simulink model "F16_fcs"  (Simulink 7.3)
settings: Solver=ode3  StartTime=0.0  StopTime=simtime  FixedStep=0.02  RelTol=1e-3
undefined symbols (not defined in the file or in its folder): alpha_trim, da_trim, del_trim, der_trim, dlef_trim, dr_trim, Earth, f16, fi_flag_Simulink, m, mlu, roll_trim, s, V_trim, WGS84, yaw_trim
libraries: simulink_extras x16, aerolibfltsims x3, aerolibtransform2 x3, simulink x2, aerolibanimutils x2, aerolibconvert2 x2, aerolibconvert x1, aerolibutil x1
settings Model: Creator=larssonneveldt  LastModifiedBy=Administrator
settings DataIOCC: SignalLoggingName=sigsOut
settings OptimizationCC: InlineInvariantSignals=on  InitFltsAndDblsToZero=on
settings DebuggingCC: SignalResolutionControl=TryResolveAllWithWarning  SolverPrmCheckMsg=none  MultiTaskDSMMsg=warning  MultiTaskCondExecSysMsg=none  StrictBusMsg=None
settings HardwareCC: TargetHWDeviceType=32-bit Generic  TargetUnknown=on  ProdEqTarget=off
settings RTWCC: IncludeERTFirstTime=on
settings GRTTargetCC: TargetFcnLib=ansi_tfl_tmw.mat

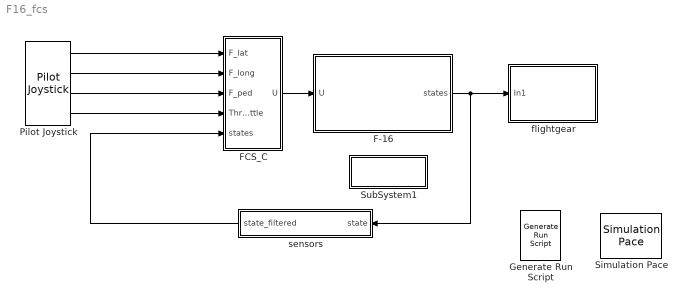
== system F16_fcs ==
  F-16 : Subsystem
      mask Display: image(imread('aerodata/f16.jpg'))
  FCS_C : Subsystem
  Generate Run Script : aerolibfltsims/Generate Run Script  DialogController=Aeroblks.DDGSource  SystemSampleTime=-1  OutputFileName=runfg.bat  FlightGearBaseDirectory=D:\Program Files\FlightGear  GeometryModelName=f16-mlu  DestinationPort=5502  AirportId=KSFO  RunwayId=10L  InitialAltitude=1000  InitialHeading=113  OffsetDistance=4.72  OffsetAzimuth=0  GenerateFile=off
  Pilot Joystick : aerolibanimutils/Pilot Joystick  JoystickID=Joystick1  OutputConfiguration=FourAxis  SampleTime=1/50
  Simulation Pace : aerolibanimutils/Simulation Pace  SimulationPace=1  SleepMode=MATLAB Thread  OutputPaceError=off  SampleTime=-1
      settings: AttributesFormatString=%<SimulationPace> sec/sec
  SubSystem1 : Subsystem
      settings: OpenFcn=edit(fullfile(cd,'F16_dyn.c'))
      mask Display: disp('F16_dyn.c');
  flightgear : Subsystem
  sensors : Subsystem
  wires:
  Pilot Joystick/1 -> FCS_C/1(F_lat)
  Pilot Joystick/2 -> FCS_C/2(F_long)
  Pilot Joystick/4 -> FCS_C/4(Throttle)
  sensors/1(state_filtered) -> FCS_C/5(states)
  F-16/1(states) -> flightgear/1(In1), sensors/1(state)
  FCS_C/1(U) -> F-16/1(U)
  Pilot Joystick/3 -> FCS_C/3(F_ped)

== system F16_fcs/F-16 ==
  U : Inport
  F-16 dynamics : S-Function  FunctionName=F16_dyn  Parameters=init_x  EnableBusSupport=off
      mask Display: image(imread('aerodata/f16.jpg'))
  LEF : Subsystem
      mask Display: port_label('output', 1, 'dlef')
  Mux : Mux  Inputs=2
  fi_flag : Constant  Value=fi_flag_Simulink  OutDataType=sfix(16)  OutScaling=2^0
  states : Outport
  wires:
  fi_flag/1 -> F-16 dynamics/3
  LEF/1("delta_lef ") -> F-16 dynamics/2
  U/1 -> F-16 dynamics/1
  F-16 dynamics/1 -> LEF/1(state), Mux/1
  F-16 dynamics/2 -> Mux/2
  Mux/1 -> states/1

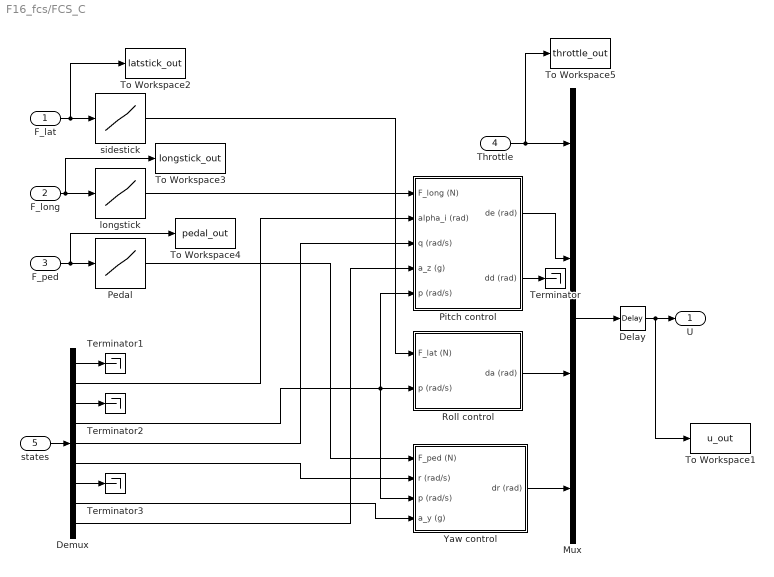
== system F16_fcs/FCS_C ==
  F_lat : Inport  OutDataType=sfix(16)  OutScaling=2^0
  F_long : Inport  Port=2  OutDataType=sfix(16)  OutScaling=2^0
  F_ped : Inport  Port=3  OutDataType=sfix(16)  OutScaling=2^0
  Throttle : Inport  Port=4  OutDataType=sfix(16)  OutScaling=2^0
  states : Inport  Port=5  OutDataType=sfix(16)  OutScaling=2^0
  Delay : TransportDelay  DelayTime=0.02
  Demux : Demux  Outputs=[2 1 3 1 1 1 4 1 1]
  Mux : Mux
  Pedal : Lookup  InputValues=[-1 -0.5 0.2 0.2 0.5 1]  Table=[-520 -70 0 0 70 520]  OutDataType=sfix(16)  OutScaling=2^0
  Pitch control : Subsystem
  Roll control : Subsystem
  Terminator{,1..3} (4 alike) : Terminator
  To Workspace1 : ToWorkspace  VariableName=u_out  SampleTime=-1  SaveFormat=Structure With Time
  To Workspace2 : ToWorkspace  VariableName=latstick_out  SampleTime=-1  SaveFormat=Structure With Time
  To Workspace3 : ToWorkspace  VariableName=longstick_out  SampleTime=-1  SaveFormat=Structure With Time
  To Workspace4 : ToWorkspace  VariableName=pedal_out  SampleTime=-1  SaveFormat=Structure With Time
  To Workspace5 : ToWorkspace  VariableName=throttle_out  SampleTime=-1  SaveFormat=Structure With Time
  Yaw control : Subsystem
  longstick : Lookup  InputValues=[-1,-0.5,-0.125,0.125,0.5,1]  Table=[-60,-20,0,0,30,160]  OutDataType=sfix(16)  OutScaling=2^0
  sidestick : Lookup  InputValues=[-1,-0.5,-0.2,0.2,0.5,1]  Table=[-80,-20,0,0,20,80]  OutDataType=sfix(16)  OutScaling=2^0
  U : Outport  OutDataType=sfix(16)  OutScaling=2^0
  wires:
  Pitch control/2(dd (rad)) -> Terminator/1
  Pitch control/1(de (rad)) -> Mux/2
  Yaw control/1(dr (rad)) -> Mux/4
  Mux/1 -> Delay/1
  Throttle/1 -> Mux/1, To Workspace5/1
  F_ped/1 -> Pedal/1, To Workspace4/1
  states/1 -> Demux/1
  Demux/1 -> Terminator1/1
  Demux/3 -> Terminator2/1
  Demux/7 -> Terminator3/1
  Demux/2 -> Pitch control/2(alpha_i (rad))
  Demux/4 -> Roll control/2(p (rad/s)), Pitch control/5(p (rad/s)), Yaw control/3(p (rad/s))
  Demux/5 -> Pitch control/3(q (rad/s))
  Demux/6 -> Yaw control/2(r (rad/s))
  F_long/1 -> longstick/1, To Workspace3/1
  F_lat/1 -> sidestick/1, To Workspace2/1
  Delay/1 -> U/1, To Workspace1/1
  Roll control/1(da (rad)) -> Mux/3
  Demux/9 -> Pitch control/4(a_z (g))
  Demux/8 -> Yaw control/4(a_y (g))
  sidestick/1 -> Roll control/1(F_lat (N))
  longstick/1 -> Pitch control/1(F_long (N))
  Pedal/1 -> Yaw control/1(F_ped (N))

== system F16_fcs/SubSystem1 ==

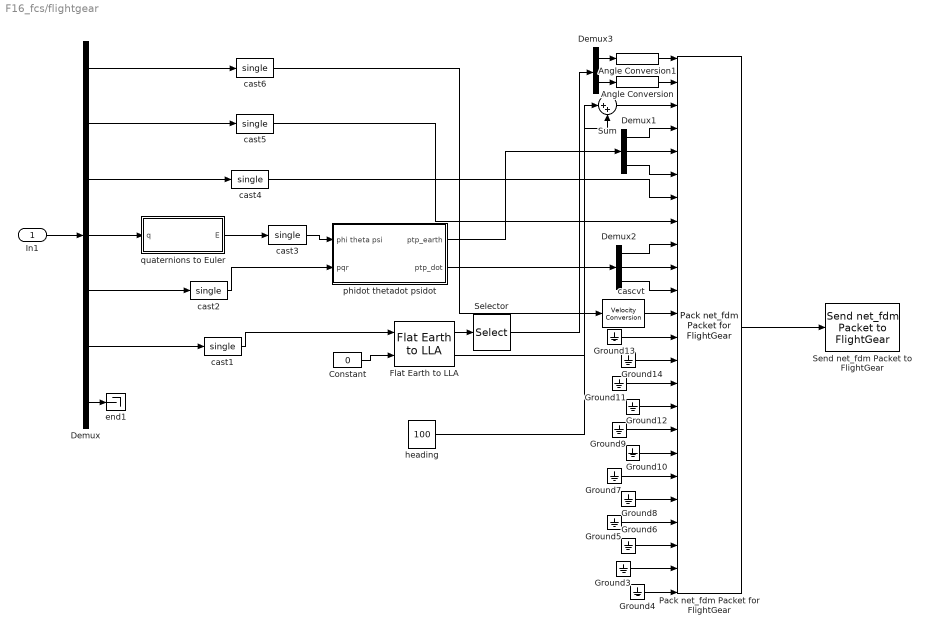
== system F16_fcs/flightgear ==
  In1 : Inport
  Angle Conversion : aerolibconvert2/Angle Conversion  SystemSampleTime=-1  IU=deg  OU=rad
  Angle Conversion1 : aerolibconvert2/Angle Conversion  SystemSampleTime=-1  IU=deg  OU=rad
  Constant : Constant  Value=0  OutDataType=sfix(16)  OutScaling=2^0
  Demux : Demux  Outputs=[1 1 1 4 3 3 3]
  Demux1 : Demux  Outputs=3
  Demux2 : Demux  Outputs=3
  Demux3 : Demux  Outputs=2
  Flat Earth to LLA : aerolibtransform2/Flat Earth to LLA  SystemSampleTime=-1  units=Metric (MKS)  ptype=Earth (WGS84)  F=1/298.257223563  R=6378137  LL0=[37.7889 -122.4778]  psi=0
  Ground{3..14} (12 alike) : Ground
  Pack net_fdm Packet for FlightGear : aerolibfltsims/Pack net_fdm Packet for FlightGear  FlightGearVersion=v0.9.10  ShowPositionAttitudeInputs=on  ShowVelocityAccelerationInputs=on  ShowControlSurfacePositionInputs=off  ShowEngineFuelInputs=off  ShowLandingGearInputs=off  ShowEnvironmentInputs=off  SampleTime=-1
  Selector : Selector  InputPortWidth=2  IndexOptions=Index vector (dialog)  Indices=[2 1]  OutputSizes=1
  Send net_fdm Packet to FlightGear : aerolibfltsims/Send net_fdm Packet to FlightGear  DestinationIpAddress=127.0.0.1  DestinationPort=5502  LocalIpPort=-1  SampleTime=-1
  Sum : Sum  Inputs=|++  OutDataType=sfix(16)  OutScaling=2^0
  cascvt : aerolibconvert/Velocity Conversion  SystemSampleTime=-1  IU=m/s  OU=kts
  cast{1..6} (6 alike) : DataTypeConversion  OutDataTypeMode=single  OutDataType=sfix(16)  OutScaling=2^0  OutDataTypeStr=single  SaturateOnIntegerOverflow=on
  end1 : Terminator
  heading : Constant  Value=100  OutDataType=sfix(16)  OutScaling=2^0
  phidot thetadot psidot : Subsystem
  quaternions to Euler : Subsystem
  wires:
  Ground3/1 -> Pack net_fdm Packet for FlightGear/23
  Ground4/1 -> Pack net_fdm Packet for FlightGear/24
  Ground5/1 -> Pack net_fdm Packet for FlightGear/21
  Ground6/1 -> Pack net_fdm Packet for FlightGear/22
  Ground7/1 -> Pack net_fdm Packet for FlightGear/19
  Ground8/1 -> Pack net_fdm Packet for FlightGear/20
  Ground9/1 -> Pack net_fdm Packet for FlightGear/17
  Ground10/1 -> Pack net_fdm Packet for FlightGear/18
  Ground11/1 -> Pack net_fdm Packet for FlightGear/15
  Ground12/1 -> Pack net_fdm Packet for FlightGear/16
  Ground13/1 -> Pack net_fdm Packet for FlightGear/13
  Ground14/1 -> Pack net_fdm Packet for FlightGear/14
  Pack net_fdm Packet for FlightGear/1 -> Send net_fdm Packet to FlightGear/1
  cascvt/1 -> Pack net_fdm Packet for FlightGear/12
  In1/1 -> Demux/1
  Demux/1 -> cast6/1
  Demux/2 -> cast5/1
  Demux1/1 -> Pack net_fdm Packet for FlightGear/4
  Demux1/3 -> Pack net_fdm Packet for FlightGear/6
  Demux/3 -> cast4/1
  Demux2/1 -> Pack net_fdm Packet for FlightGear/9
  Demux2/2 -> Pack net_fdm Packet for FlightGear/10
  Demux/5 -> cast2/1
  Demux2/3 -> Pack net_fdm Packet for FlightGear/11
  Demux1/2 -> Pack net_fdm Packet for FlightGear/5
  phidot thetadot psidot/1(ptp_earth) -> Demux1/1
  phidot thetadot psidot/2(ptp_dot) -> Demux2/1
  Demux/6 -> cast1/1
  Constant/1 -> Flat Earth to LLA/2
  Flat Earth to LLA/1 -> Selector/1
  Selector/1 -> Demux3/1
  Demux3/1 -> Angle Conversion1/1
  Demux3/2 -> Angle Conversion/1
  cast1/1 -> Flat Earth to LLA/1
  cast2/1 -> phidot thetadot psidot/2(pqr)
  cast3/1 -> phidot thetadot psidot/1(phi theta psi)
  cast4/1 -> Pack net_fdm Packet for FlightGear/7
  cast5/1 -> Pack net_fdm Packet for FlightGear/8
  cast6/1 -> cascvt/1
  Flat Earth to LLA/2 -> Sum/1
  Sum/1 -> Pack net_fdm Packet for FlightGear/3
  Angle Conversion/1 -> Pack net_fdm Packet for FlightGear/2
  Angle Conversion1/1 -> Pack net_fdm Packet for FlightGear/1
  heading/1 -> Sum/2
  quaternions to Euler/1(E) -> cast3/1
  Demux/4 -> quaternions to Euler/1(q)
  Demux/7 -> end1/1

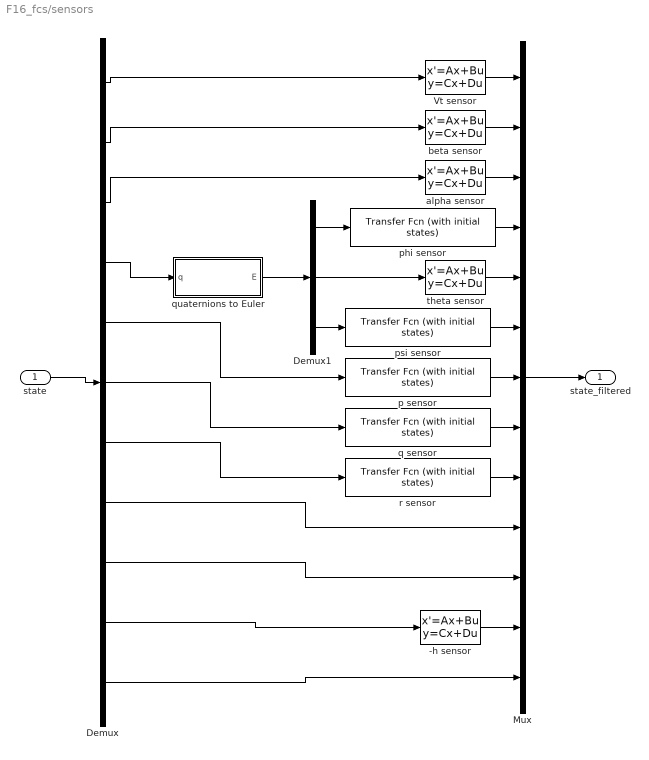
== system F16_fcs/sensors ==
  state : Inport
  -h sensor : StateSpace  A=-50  B=50  D=0  X0=alpha_trim
  Demux : Demux  Outputs=[ones(1,3) 4 ones(1,6) 3]
  Demux1 : Demux  Outputs=3
  Mux : Mux  Inputs=[ones(1,12) 3]
  Vt sensor : StateSpace  A=-50  B=50  D=0  X0=V_trim
  alpha sensor : StateSpace  A=-50  B=50  D=0  X0=alpha_trim
  beta sensor : StateSpace  A=-50  B=50  D=0
  p sensor : simulink_extras/Additional Linear/Transfer Fcn (with initial states)  SystemSampleTime=-1  N=[0.0001903 0.005346 1]  D=[0.0004942 0.03082 1]  X0=[0 0]
  phi sensor : simulink_extras/Additional Linear/Transfer Fcn (with initial states)  SystemSampleTime=-1  N=[1]  D=[0.00104 0.0323 1]  X0=[0 0]
  psi sensor : simulink_extras/Additional Linear/Transfer Fcn (with initial states)  SystemSampleTime=-1  N=[1]  D=[0.00104 0.0323 1]  X0=[0 0]
  q sensor : simulink_extras/Additional Linear/Transfer Fcn (with initial states)  SystemSampleTime=-1  N=[0.0001903 0.005346 1]  D=[0.0004942 0.03082 1]  X0=[0 0]
  quaternions to Euler : Subsystem
  r sensor : simulink_extras/Additional Linear/Transfer Fcn (with initial states)  SystemSampleTime=-1  N=[0.0001903 0.005346 1]  D=[0.0004942 0.03082 1]  X0=[0 0]
  theta sensor : StateSpace  A=-50  B=50  D=0  X0=alpha_trim
  state_filtered : Outport
  wires:
  Mux/1 -> state_filtered/1
  state/1 -> Demux/1
  r sensor/1 -> Mux/9
  q sensor/1 -> Mux/8
  p sensor/1 -> Mux/7
  psi sensor/1 -> Mux/6
  phi sensor/1 -> Mux/4
  alpha sensor/1 -> Mux/3
  beta sensor/1 -> Mux/2
  Vt sensor/1 -> Mux/1
  Demux1/1 -> phi sensor/1
  Demux1/2 -> theta sensor/1
  Demux1/3 -> psi sensor/1
  -h sensor/1 -> Mux/12
  quaternions to Euler/1(E) -> Demux1/1
  theta sensor/1 -> Mux/5
  Demux/1 -> Vt sensor/1
  Demux/2 -> beta sensor/1
  Demux/3 -> alpha sensor/1
  Demux/4 -> quaternions to Euler/1(q)
  Demux/5 -> p sensor/1
  Demux/6 -> q sensor/1
  Demux/7 -> r sensor/1
  Demux/8 -> Mux/10
  Demux/9 -> Mux/11
  Demux/10 -> -h sensor/1
  Demux/11 -> Mux/13

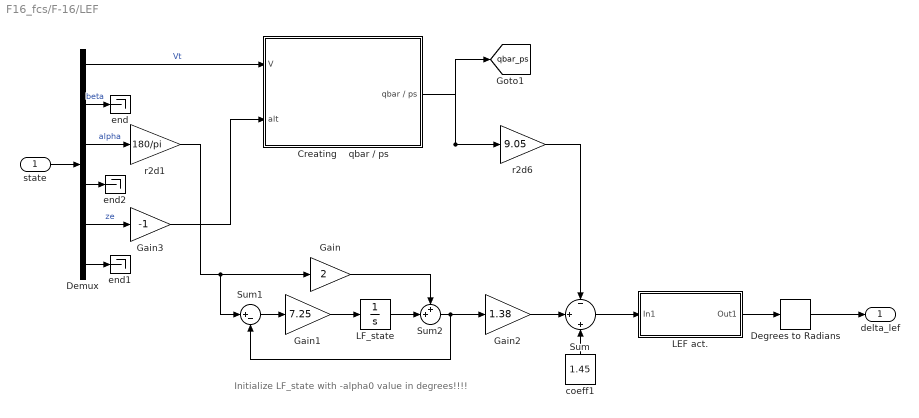
== system F16_fcs/F-16/LEF ==
  note: Initialize LF_state with -alpha0 value in degrees!!!!
  state : Inport  OutDataType=sfix(16)  OutScaling=2^0
  Creating    qbar / ps : Subsystem
  Degrees to Radians : simulink_extras/Transformations/Degrees to Radians  SystemSampleTime=-1
  Demux : Demux  Outputs=[1 1 1 9 1 1]
  Gain : Gain  Gain=2  ParameterDataType=sfix(16)  ParameterScaling=2^0  OutDataType=sfix(16)  OutScaling=2^0  SaturateOnIntegerOverflow=on  OutDataTypeStr=Inherit: Same as input  ParamDataTypeStr=Inherit: Same as input
  Gain1 : Gain  Gain=7.25  ParameterDataType=sfix(16)  ParameterScaling=2^0  OutDataType=sfix(16)  OutScaling=2^0  SaturateOnIntegerOverflow=on  OutDataTypeStr=Inherit: Same as input  ParamDataTypeStr=Inherit: Same as input
  Gain2 : Gain  Gain=1.38  ParameterDataType=sfix(16)  ParameterScaling=2^0  OutDataType=sfix(16)  OutScaling=2^0  SaturateOnIntegerOverflow=on  OutDataTypeStr=Inherit: Same as input  ParamDataTypeStr=Inherit: Same as input
  Gain3 : Gain  Gain=-1  ParameterDataType=sfix(16)  ParameterScaling=2^0  OutDataType=sfix(16)  OutScaling=2^0  SaturateOnIntegerOverflow=on  OutDataTypeStr=Inherit: Same as input  ParamDataTypeStr=Inherit: Same as input
  LEF act. : Subsystem
  LF_state : Integrator  InitialCondition=-alpha_trim*180/pi
  Sum : Sum  Inputs=-|+|+  OutDataType=sfix(16)  OutScaling=2^0  SaturateOnIntegerOverflow=on  InputSameDT=on  OutDataTypeStr=Inherit: Same as first input
  Sum1 : Sum  Inputs=|+-  OutDataType=sfix(16)  OutScaling=2^0  SaturateOnIntegerOverflow=on  InputSameDT=on  OutDataTypeStr=Inherit: Same as first input
  Sum2 : Sum  Inputs=++|  OutDataType=sfix(16)  OutScaling=2^0  SaturateOnIntegerOverflow=on  InputSameDT=on  OutDataTypeStr=Inherit: Same as first input
  coeff1 : Constant  Value=1.45  OutDataType=sfix(16)  OutScaling=2^0
  end : Terminator
  end1 : Terminator
  end2 : Terminator
  r2d1 : Gain  Gain=180/pi  ParameterDataType=sfix(16)  ParameterScaling=2^0  OutDataType=sfix(16)  OutScaling=2^0  SaturateOnIntegerOverflow=on  OutDataTypeStr=Inherit: Same as input  ParamDataTypeStr=Inherit: Same as input
  r2d6 : Gain  Gain=9.05  ParameterDataType=sfix(16)  ParameterScaling=2^0  OutDataType=sfix(16)  OutScaling=2^0  SaturateOnIntegerOverflow=on  OutDataTypeStr=Inherit: Same as input  ParamDataTypeStr=Inherit: Same as input
  "delta_lef " : Outport  OutDataType=sfix(16)  OutScaling=2^0
  tag scope: qbar_ps=global
  wires:
  Degrees to Radians/1 -> "delta_lef "/1
  Gain3/1 -> Creating    qbar / ps/2(alt)
  LEF act./1(Out1) -> Degrees to Radians/1
  Sum/1 -> LEF act./1(In1)
  state/1 -> Demux/1
  Sum1/1 -> Gain1/1
  Gain1/1 -> LF_state/1
  Gain/1 -> Sum2/1
  Gain2/1 -> Sum/2
  coeff1/1 -> Sum/3
  Sum2/1 -> Sum1/2, Gain2/1
  LF_state/1 -> Sum2/2
  r2d1/1 -> Sum1/1, Gain/1
  Creating    qbar / ps/1(qbar / ps) -> r2d6/1, [qbar_ps]
  r2d6/1 -> Sum/1
  Demux/1 -> Creating    qbar / ps/1(V)  "Vt"
  Demux/2 -> end/1  "beta"
  Demux/3 -> r2d1/1  "alpha"
  Demux/4 -> end2/1
  Demux/5 -> Gain3/1  "ze"
  Demux/6 -> end1/1

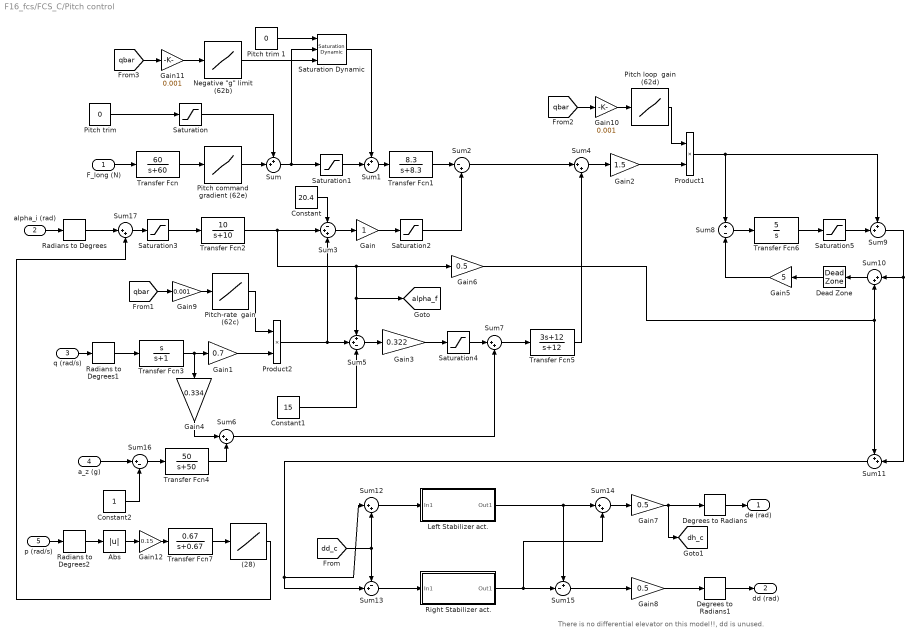
== system F16_fcs/FCS_C/Pitch control ==
  note: There is no differential elevator on this model!!, dd is unused.
  F_long (N) : Inport  OutDataType=sfix(16)  OutScaling=2^0
  alpha_i (rad) : Inport  Port=2  OutDataType=sfix(16)  OutScaling=2^0
  q (rad/s) : Inport  Port=3  OutDataType=sfix(16)  OutScaling=2^0
  a_z (g) : Inport  Port=4  OutDataType=sfix(16)  OutScaling=2^0
  p (rad/s) : Inport  Port=5  OutDataType=sfix(16)  OutScaling=2^0
  " (28)" : Lookup  InputValues=[0 3 8.4 50]  Table=[0 0 5.4 5.4]  OutDataType=sfix(16)  OutScaling=2^0
  Abs : Abs
  Constant : Constant  Value=20.4  OutDataType=sfix(16)  OutScaling=2^0
  Constant1 : Constant  Value=15  OutDataType=sfix(16)  OutScaling=2^0
  Constant2 : Constant  OutDataType=sfix(16)  OutScaling=2^0
  Dead Zone : DeadZone  LowerValue=-25  UpperValue=25  SaturateOnIntegerOverflow=on
  Degrees to Radians : simulink_extras/Transformations/Degrees to Radians  SystemSampleTime=-1
  Degrees to Radians1 : simulink_extras/Transformations/Degrees to Radians  SystemSampleTime=-1
  Gain : Gain  ParameterDataType=sfix(16)  ParameterScaling=2^0  OutDataType=sfix(16)  OutScaling=2^0
  Gain1 : Gain  Gain=0.7  ParameterDataType=sfix(16)  ParameterScaling=2^0  OutDataType=sfix(16)  OutScaling=2^0
  Gain10 : Gain  Gain=0.001  ParameterDataType=sfix(16)  ParameterScaling=2^0  OutDataType=sfix(16)  OutScaling=2^0
  Gain11 : Gain  Gain=0.001  ParameterDataType=sfix(16)  ParameterScaling=2^0  OutDataType=sfix(16)  OutScaling=2^0
  Gain12 : Gain  Gain=0.15  ParameterDataType=sfix(16)  ParameterScaling=2^0  OutDataType=sfix(16)  OutScaling=2^0
  Gain2 : Gain  Gain=1.5  ParameterDataType=sfix(16)  ParameterScaling=2^0  OutDataType=sfix(16)  OutScaling=2^0
  Gain3 : Gain  Gain=0.322  ParameterDataType=sfix(16)  ParameterScaling=2^0  OutDataType=sfix(16)  OutScaling=2^0
  Gain4 : Gain  Gain=0.334  ParameterDataType=sfix(16)  ParameterScaling=2^0  OutDataType=sfix(16)  OutScaling=2^0
  Gain5 : Gain  Gain=5  ParameterDataType=sfix(16)  ParameterScaling=2^0  OutDataType=sfix(16)  OutScaling=2^0
  Gain6 : Gain  Gain=0.5  ParameterDataType=sfix(16)  ParameterScaling=2^0  OutDataType=sfix(16)  OutScaling=2^0
  Gain7 : Gain  Gain=0.5  ParameterDataType=sfix(16)  ParameterScaling=2^0  OutDataType=sfix(16)  OutScaling=2^0
  Gain8 : Gain  Gain=0.5  ParameterDataType=sfix(16)  ParameterScaling=2^0  OutDataType=sfix(16)  OutScaling=2^0
  Gain9 : Gain  Gain=0.001  ParameterDataType=sfix(16)  ParameterScaling=2^0  OutDataType=sfix(16)  OutScaling=2^0
  Left Stabilizer act. : Subsystem
      mask Display:
      | port_label('output', 1, 'dhr')
      | port_label('input', 1, 'dhr_c')
  "Negative \"g\" limit (62b)" : Lookup  InputValues=[0,1.75,8.75,10]  Table=[-1,-1,-4,-4]  OutDataType=sfix(16)  OutScaling=2^0
  Pitch command gradient (62e) : Lookup  InputValues=[-80, -30, -7.5, 7.5, 30, 160]  Table=[-4,-0.75, 0, 0, 0.5, 10]  OutDataType=sfix(16)  OutScaling=2^0
  Pitch loop  gain (62d) : Lookup  InputValues=[0,12,43.3,56]  Table=[1,1,0.4,0.4]  OutDataType=sfix(16)  OutScaling=2^0
  "Pitch trim " : Constant  Value=0  OutDataType=sfix(16)  OutScaling=2^0
  Pitch trim 1 : Constant  Value=0  OutDataType=sfix(16)  OutScaling=2^0
  Pitch-rate  gain (62c) : Lookup  InputValues=[0,5, 15,20]  Table=[1,1,0.3,0.3]  OutDataType=sfix(16)  OutScaling=2^0
  Product1 : Product  OutDataType=sfix(16)  OutScaling=2^0  RndMeth=Zero
  Product2 : Product  OutDataType=sfix(16)  OutScaling=2^0  RndMeth=Zero
  Radians to Degrees : simulink_extras/Transformations/Radians to Degrees  SystemSampleTime=-1
  Radians to Degrees1 : simulink_extras/Transformations/Radians to Degrees  SystemSampleTime=-1
  Radians to Degrees2 : simulink_extras/Transformations/Radians to Degrees  SystemSampleTime=-1
  Right Stabilizer act. : Subsystem
      mask Display:
      | port_label('output', 1, 'dhl')
      | port_label('input', 1, 'dhl_c')
  Saturation : Saturate  UpperLimit=2.4  LowerLimit=-2.4
  Saturation Dynamic : simulink/Discontinuities/Saturation Dynamic  SystemSampleTime=-1  OutMin=[]  OutMax=[]  OutDataTypeStr=Inherit: Same as second input  OutDataType=sfix(16)  OutScaling=2^-10  DoSatur=off
  Saturation1 : Saturate  UpperLimit=8  LowerLimit=0
  Saturation2 : Saturate  UpperLimit=Inf  LowerLimit=0
  Saturation3 : Saturate  UpperLimit=30  LowerLimit=-5
  Saturation4 : Saturate  UpperLimit=Inf  LowerLimit=0
  Saturation5 : Saturate  UpperLimit=25  LowerLimit=-25
  Sum{,1,9,11} (4 alike) : Sum  Inputs=++|  OutDataType=sfix(16)  OutScaling=2^0
  Sum{4,6..7,10,12,14,17} (7 alike) : Sum  Inputs=|++  OutDataType=sfix(16)  OutScaling=2^0
  Sum13 : Sum  Inputs=-+|  OutDataType=sfix(16)  OutScaling=2^0
  Sum15 : Sum  Inputs=+-|  OutDataType=sfix(16)  OutScaling=2^0
  Sum16 : Sum  Inputs=|+-  OutDataType=sfix(16)  OutScaling=2^0
  Sum2 : Sum  Inputs=|-+  OutDataType=sfix(16)  OutScaling=2^0
  Sum3 : Sum  Inputs=-++  OutDataType=sfix(16)  OutScaling=2^0
  Sum5 : Sum  Inputs=++-  OutDataType=sfix(16)  OutScaling=2^0
  Sum8 : Sum  Inputs=+|-  OutDataType=sfix(16)  OutScaling=2^0
  Transfer Fcn : TransferFcn  Numerator=60  Denominator=[1 60]
  Transfer Fcn1 : TransferFcn  Numerator=8.3  Denominator=[1 8.3]
  Transfer Fcn2 : TransferFcn  Numerator=10  Denominator=[1 10]
  Transfer Fcn3 : TransferFcn  Numerator=[1 0]  Denominator=[1 1]
  Transfer Fcn4 : TransferFcn  Numerator=50  Denominator=[1 50]
  Transfer Fcn5 : TransferFcn  Numerator=[3 12]  Denominator=[1 12]
  Transfer Fcn6 : TransferFcn  Numerator=5  Denominator=[1 0]
  Transfer Fcn7 : TransferFcn  Numerator=0.67  Denominator=[1 0.67]
  de (rad) : Outport  OutDataType=sfix(16)  OutScaling=2^0
  dd (rad) : Outport  Port=2  OutDataType=sfix(16)  OutScaling=2^0
  tag scope: alpha_f=global, dh_c=global
  wires:
  F_long (N)/1 -> Transfer Fcn/1
  Transfer Fcn/1 -> Pitch command gradient (62e)/1
  Pitch command gradient (62e)/1 -> Sum/2
  Sum/1 -> Saturation1/1, Saturation Dynamic/2
  Saturation1/1 -> Sum1/2
  Sum1/1 -> Transfer Fcn1/1
  Transfer Fcn1/1 -> Sum2/1
  Saturation2/1 -> Sum2/2
  Gain/1 -> Saturation2/1
  Sum3/1 -> Gain/1
  Constant/1 -> Sum3/1
  Transfer Fcn2/1 -> Sum3/2, Gain6/1, Sum5/1, [alpha_f]
  Saturation3/1 -> Transfer Fcn2/1
  q (rad/s)/1 -> Radians to Degrees1/1
  Transfer Fcn3/1 -> Gain1/1, Gain4/1
  Gain1/1 -> Product2/2
  Sum2/1 -> Sum4/1
  Product2/1 -> Sum3/3, Sum5/2
  Constant1/1 -> Sum5/3
  Sum5/1 -> Gain3/1
  Gain3/1 -> Saturation4/1
  Transfer Fcn4/1 -> Sum6/2
  Gain4/1 -> Sum6/1
  Sum6/1 -> Sum7/2
  Saturation4/1 -> Sum7/1
  Sum7/1 -> Transfer Fcn5/1
  Transfer Fcn5/1 -> Sum4/2
  Sum4/1 -> Gain2/1
  Gain2/1 -> Product1/2
  Transfer Fcn6/1 -> Saturation5/1
  Sum8/1 -> Transfer Fcn6/1
  Product1/1 -> Sum8/1, Sum9/1
  Dead Zone/1 -> Gain5/1
  Gain5/1 -> Sum8/2
  Saturation5/1 -> Sum9/2
  Sum10/1 -> Dead Zone/1
  Gain6/1 -> Sum11/1, Sum10/2
  Sum9/1 -> Sum11/2, Sum10/1
  Sum11/1 -> Sum12/1, Sum13/2
  [dd_c] -> Sum12/2, Sum13/1
  Sum13/1 -> Right Stabilizer act./1(In1)
  Sum12/1 -> Left Stabilizer act./1(In1)
  Left Stabilizer act./1(Out1) -> Sum15/1, Sum14/1
  Right Stabilizer act./1(Out1) -> Sum15/2, Sum14/2
  Sum14/1 -> Gain7/1
  Sum15/1 -> Gain8/1
  Gain8/1 -> Degrees to Radians1/1
  Gain7/1 -> [dh_c], Degrees to Radians/1
  a_z (g)/1 -> Sum16/1
  Sum16/1 -> Transfer Fcn4/1
  Gain11/1 -> "Negative \"g\" limit (62b)"/1
  Gain10/1 -> Pitch loop  gain (62d)/1
  Pitch loop  gain (62d)/1 -> Product1/1
  [qbar] -> Gain9/1
  Gain9/1 -> Pitch-rate  gain (62c)/1
  Pitch-rate  gain (62c)/1 -> Product2/1
  Saturation/1 -> Sum/1
  "Pitch trim "/1 -> Saturation/1
  p (rad/s)/1 -> Radians to Degrees2/1
  Abs/1 -> Gain12/1
  Gain12/1 -> Transfer Fcn7/1
  Transfer Fcn7/1 -> " (28)"/1
  alpha_i (rad)/1 -> Radians to Degrees/1
  Sum17/1 -> Saturation3/1
  Constant2/1 -> Sum16/2
  [qbar] -> Gain11/1
  [qbar] -> Gain10/1
  Degrees to Radians/1 -> de (rad)/1
  Degrees to Radians1/1 -> dd (rad)/1
  " (28)"/1 -> Sum17/2
  Radians to Degrees/1 -> Sum17/1
  Radians to Degrees1/1 -> Transfer Fcn3/1
  Radians to Degrees2/1 -> Abs/1
  "Negative \"g\" limit (62b)"/1 -> Saturation Dynamic/3
  Pitch trim 1/1 -> Saturation Dynamic/1
  Saturation Dynamic/1 -> Sum1/1

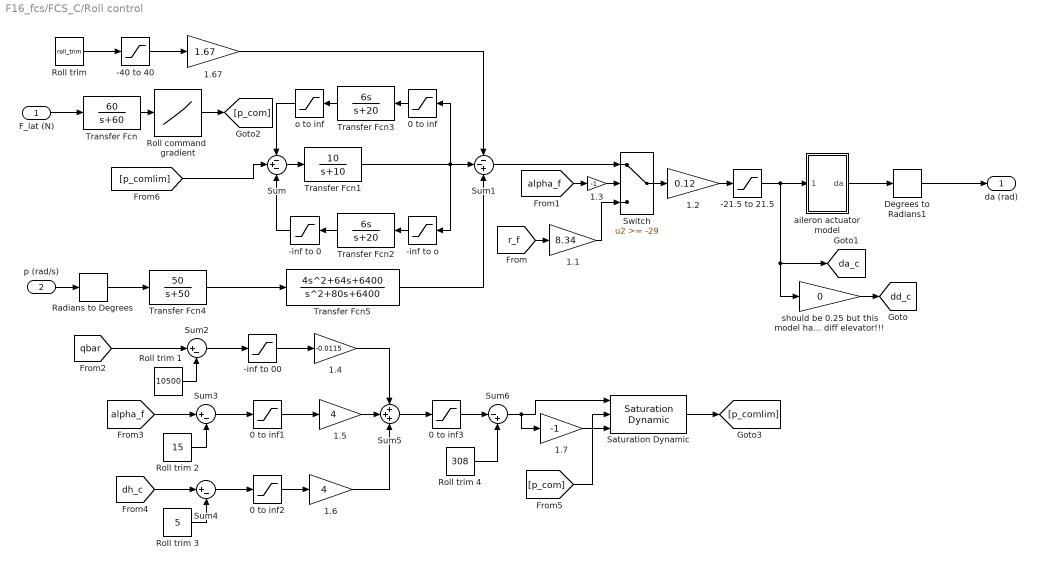
== system F16_fcs/FCS_C/Roll control ==
  F_lat (N) : Inport  OutDataType=sfix(16)  OutScaling=2^0
  p (rad/s) : Inport  Port=2  OutDataType=sfix(16)  OutScaling=2^0
  -21.5 to 21.5 : Saturate  UpperLimit=21.5  LowerLimit=-21.5
  -40 to 40 : Saturate  UpperLimit=40  LowerLimit=-40
  -inf to 0 : Saturate  UpperLimit=0  LowerLimit=-inf
  -inf to 00 : Saturate  UpperLimit=0  LowerLimit=-inf
  -inf to o : Saturate  UpperLimit=0  LowerLimit=-inf  LinearizeAsGain=off
  0 to inf : Saturate  UpperLimit=inf  LowerLimit=0
  0 to inf1 : Saturate  UpperLimit=inf  LowerLimit=0
  0 to inf2 : Saturate  UpperLimit=inf  LowerLimit=0
  0 to inf3 : Saturate  UpperLimit=228  LowerLimit=0
  1.1 : Gain  Gain=8.34  ParameterDataType=sfix(16)  ParameterScaling=2^0  OutDataType=sfix(16)  OutScaling=2^0
  1.2 : Gain  Gain=0.12  ParameterDataType=sfix(16)  ParameterScaling=2^0  OutDataType=sfix(16)  OutScaling=2^0
  1.3 : Gain  Gain=-1  ParameterDataType=sfix(16)  ParameterScaling=2^0  OutDataType=sfix(16)  OutScaling=2^0
  1.4 : Gain  Gain=-0.0115  ParameterDataType=sfix(16)  ParameterScaling=2^0  OutDataType=sfix(16)  OutScaling=2^0
  1.5 : Gain  Gain=4  ParameterDataType=sfix(16)  ParameterScaling=2^0  OutDataType=sfix(16)  OutScaling=2^0
  1.6 : Gain  Gain=4  ParameterDataType=sfix(16)  ParameterScaling=2^0  OutDataType=sfix(16)  OutScaling=2^0
  1.67 : Gain  Gain=1.67  ParameterDataType=sfix(16)  ParameterScaling=2^0  OutDataType=sfix(16)  OutScaling=2^0
  1.7 : Gain  Gain=-1  ParameterDataType=sfix(16)  ParameterScaling=2^0  OutDataType=sfix(16)  OutScaling=2^0
  Degrees to Radians1 : simulink_extras/Transformations/Degrees to Radians  SystemSampleTime=-1
  Radians to Degrees : simulink_extras/Transformations/Radians to Degrees  SystemSampleTime=-1
  Roll command  gradient : Lookup  InputValues=[-79 -49 -26 -6 6 26 49 79]  Table=[-335 -80 -20 0 0 20 80 335]  OutDataType=sfix(16)  OutScaling=2^0
  "Roll trim " : Constant  Value=roll_trim  OutDataType=sfix(16)  OutScaling=2^0
  Roll trim 1 : Constant  Value=10500  OutDataType=sfix(16)  OutScaling=2^0
  Roll trim 2 : Constant  Value=15  OutDataType=sfix(16)  OutScaling=2^0
  Roll trim 3 : Constant  Value=5  OutDataType=sfix(16)  OutScaling=2^0
  Roll trim 4 : Constant  Value=308  OutDataType=sfix(16)  OutScaling=2^0
  Saturation Dynamic : simulink/Discontinuities/Saturation Dynamic  SystemSampleTime=-1  OutMin=[]  OutMax=[]  OutDataTypeStr=Inherit: Same as second input  OutDataType=sfix(16)  OutScaling=2^-10  DoSatur=off
  Sum : Sum  Inputs=-+-  OutDataType=sfix(16)  OutScaling=2^0
  Sum1 : Sum  Inputs=--+  OutDataType=sfix(16)  OutScaling=2^0
  Sum2 : Sum  Inputs=|+-  OutDataType=sfix(16)  OutScaling=2^0
  Sum3 : Sum  Inputs=|+-  OutDataType=sfix(16)  OutScaling=2^0
  Sum4 : Sum  Inputs=|+-  OutDataType=sfix(16)  OutScaling=2^0
  Sum5 : Sum  Inputs=+++  OutDataType=sfix(16)  OutScaling=2^0
  Sum6 : Sum  Inputs=|-+  OutDataType=sfix(16)  OutScaling=2^0
  Switch : Switch  Threshold=-29
  Transfer Fcn : TransferFcn  Numerator=60  Denominator=[1 60]
  Transfer Fcn1 : TransferFcn  Numerator=10  Denominator=[1 10]
  Transfer Fcn2 : TransferFcn  Numerator=[6 0]  Denominator=[1 20]
  Transfer Fcn3 : TransferFcn  Numerator=[6 0]  Denominator=[1 20]
  Transfer Fcn4 : TransferFcn  Numerator=50  Denominator=[1 50]
  Transfer Fcn5 : TransferFcn  Numerator=[4 64 6400]  Denominator=[1 80 6400]
  aileron actuator model : Subsystem
  o to inf : Saturate  UpperLimit=inf  LowerLimit=0
  should be 0.25 but this model has no diff elevator!!! : Gain  Gain=0  ParameterDataType=sfix(16)  ParameterScaling=2^0  OutDataType=sfix(16)  OutScaling=2^0
  da (rad) : Outport  OutDataType=sfix(16)  OutScaling=2^0
  tag scope: da_c=global, dd_c=global
  wires:
  "Roll trim "/1 -> -40 to 40/1
  -40 to 40/1 -> 1.67/1
  F_lat (N)/1 -> Transfer Fcn/1
  Transfer Fcn/1 -> Roll command  gradient/1
  Sum/1 -> Transfer Fcn1/1
  -inf to o/1 -> Transfer Fcn2/1
  Transfer Fcn2/1 -> -inf to 0/1
  -inf to 0/1 -> Sum/3
  0 to inf/1 -> Transfer Fcn3/1
  Transfer Fcn3/1 -> o to inf/1
  o to inf/1 -> Sum/1
  1.67/1 -> Sum1/1
  Transfer Fcn1/1 -> -inf to o/1, 0 to inf/1, Sum1/2
  p (rad/s)/1 -> Radians to Degrees/1
  Transfer Fcn4/1 -> Transfer Fcn5/1
  Transfer Fcn5/1 -> Sum1/3
  Sum1/1 -> Switch/1
  [r_f] -> 1.1/1
  Switch/1 -> 1.2/1
  1.1/1 -> Switch/3
  1.2/1 -> -21.5 to 21.5/1
  -21.5 to 21.5/1 -> aileron actuator model/1(da_c), should be 0.25 but this model has no diff elevator!!!/1, [da_c]
  aileron actuator model/1(da) -> Degrees to Radians1/1
  should be 0.25 but this model has no diff elevator!!!/1 -> [dd_c]
  [alpha_f] -> 1.3/1
  1.3/1 -> Switch/2
  Roll trim 1/1 -> Sum2/2
  [alpha_f] -> Sum3/1
  Roll trim 2/1 -> Sum3/2
  [dh_c] -> Sum4/1
  Roll trim 3/1 -> Sum4/2
  Sum3/1 -> 0 to inf1/1
  Sum4/1 -> 0 to inf2/1
  Sum2/1 -> -inf to 00/1
  -inf to 00/1 -> 1.4/1
  0 to inf1/1 -> 1.5/1
  0 to inf2/1 -> 1.6/1
  1.4/1 -> Sum5/1
  1.5/1 -> Sum5/2
  1.6/1 -> Sum5/3
  Sum5/1 -> 0 to inf3/1
  0 to inf3/1 -> Sum6/1
  Roll trim 4/1 -> Sum6/2
  Sum6/1 -> Saturation Dynamic/1, 1.7/1
  1.7/1 -> Saturation Dynamic/3
  Roll command  gradient/1 -> [p_com]
  [p_com] -> Saturation Dynamic/2
  Saturation Dynamic/1 -> [p_comlim]
  [p_comlim] -> Sum/2
  [qbar] -> Sum2/1
  Degrees to Radians1/1 -> da (rad)/1
  Radians to Degrees/1 -> Transfer Fcn4/1

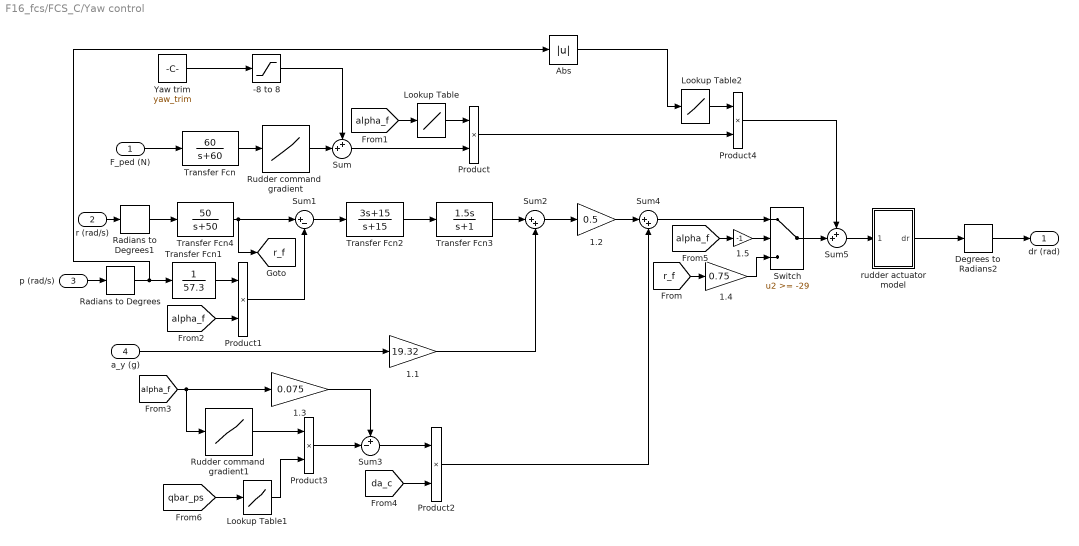
== system F16_fcs/FCS_C/Yaw control ==
  F_ped (N) : Inport  OutDataType=sfix(16)  OutScaling=2^0
  r (rad/s) : Inport  Port=2  OutDataType=sfix(16)  OutScaling=2^0
  p (rad/s) : Inport  Port=3  OutDataType=sfix(16)  OutScaling=2^0
  a_y (g) : Inport  Port=4  OutDataType=sfix(16)  OutScaling=2^0
  -8 to 8 : Saturate  UpperLimit=8  LowerLimit=-8
  1.1 : Gain  Gain=19.32  ParameterDataType=sfix(16)  ParameterScaling=2^0  OutDataType=sfix(16)  OutScaling=2^0
  1.2 : Gain  Gain=0.5  ParameterDataType=sfix(16)  ParameterScaling=2^0  OutDataType=sfix(16)  OutScaling=2^0
  1.3 : Gain  Gain=0.075  ParameterDataType=sfix(16)  ParameterScaling=2^0  OutDataType=sfix(16)  OutScaling=2^0
  1.4 : Gain  Gain=0.75  ParameterDataType=sfix(16)  ParameterScaling=2^0  OutDataType=sfix(16)  OutScaling=2^0
  1.5 : Gain  Gain=-1  ParameterDataType=sfix(16)  ParameterScaling=2^0  OutDataType=sfix(16)  OutScaling=2^0
  Abs : Abs
  Degrees to Radians2 : simulink_extras/Transformations/Degrees to Radians  SystemSampleTime=-1
  Lookup Table : Lookup  InputValues=[-90 20 30 90]  Table=[1 1 0 0]  OutDataType=sfix(16)  OutScaling=2^0
  Lookup Table1 : Lookup  InputValues=[-10 0.187 1.129 100]  Table=[0 0 1 1]  OutDataType=sfix(16)  OutScaling=2^0
  Lookup Table2 : Lookup  InputValues=[0 20 40 100]  Table=[1 1 0 0]  OutDataType=sfix(16)  OutScaling=2^0
  Product{,1..4} (5 alike) : Product  OutDataType=sfix(16)  OutScaling=2^0  RndMeth=Zero
  Radians to Degrees : simulink_extras/Transformations/Radians to Degrees  SystemSampleTime=-1
  Radians to Degrees1 : simulink_extras/Transformations/Radians to Degrees  SystemSampleTime=-1
  Rudder command  gradient : Lookup  InputValues=[-520 -70 70 520]  Table=[-34 0 0 34]  OutDataType=sfix(16)  OutScaling=2^0
  Rudder command  gradient1 : Lookup  InputValues=[-90 -10 0 10 90]  Table=[0 0 1 0 0]  OutDataType=sfix(16)  OutScaling=2^0
  Sum : Sum  Inputs=++|  OutDataType=sfix(16)  OutScaling=2^0
  Sum1 : Sum  Inputs=|+-  OutDataType=sfix(16)  OutScaling=2^0
  Sum2 : Sum  Inputs=|++  OutDataType=sfix(16)  OutScaling=2^0
  Sum3 : Sum  Inputs=+-|  OutDataType=sfix(16)  OutScaling=2^0
  Sum4 : Sum  Inputs=|++  OutDataType=sfix(16)  OutScaling=2^0
  Sum5 : Sum  Inputs=++|  OutDataType=sfix(16)  OutScaling=2^0
  Switch : Switch  Threshold=-29
  Transfer Fcn : TransferFcn  Numerator=60  Denominator=[1 60]
  Transfer Fcn1 : TransferFcn  Numerator=1  Denominator=57.3
  Transfer Fcn2 : TransferFcn  Numerator=[3 15]  Denominator=[1 15]
  Transfer Fcn3 : TransferFcn  Numerator=[1.5 0]  Denominator=[1 1]
  Transfer Fcn4 : TransferFcn  Numerator=50  Denominator=[1 50]
  Yaw trim : Constant  Value=yaw_trim  OutDataType=sfix(16)  OutScaling=2^0
  rudder actuator model : Subsystem
  dr (rad) : Outport  OutDataType=sfix(16)  OutScaling=2^0
  tag scope: r_f=global
  wires:
  Yaw trim/1 -> -8 to 8/1
  F_ped (N)/1 -> Transfer Fcn/1
  r (rad/s)/1 -> Radians to Degrees1/1
  p (rad/s)/1 -> Radians to Degrees/1
  Transfer Fcn/1 -> Rudder command  gradient/1
  Rudder command  gradient/1 -> Sum/2
  -8 to 8/1 -> Sum/1
  [alpha_f] -> Lookup Table/1
  Sum/1 -> Product/2
  Lookup Table/1 -> Product/1
  Transfer Fcn4/1 -> Sum1/1, [r_f]
  Transfer Fcn1/1 -> Product1/1
  [alpha_f] -> Product1/2
  Product1/1 -> Sum1/2
  Sum1/1 -> Transfer Fcn2/1
  Transfer Fcn2/1 -> Transfer Fcn3/1
  a_y (g)/1 -> 1.1/1
  Transfer Fcn3/1 -> Sum2/1
  1.1/1 -> Sum2/2
  Sum2/1 -> 1.2/1
  [alpha_f] -> 1.3/1, Rudder command  gradient1/1
  1.3/1 -> Sum3/1
  Sum3/1 -> Product2/1
  [da_c] -> Product2/2
  1.2/1 -> Sum4/1
  Product2/1 -> Sum4/2
  [alpha_f] -> 1.5/1
  [r_f] -> 1.4/1
  1.4/1 -> Switch/3
  Sum4/1 -> Switch/1
  Switch/1 -> Sum5/2
  Product/1 -> Product4/2
  Sum5/1 -> rudder actuator model/1(dr_c)
  rudder actuator model/1(dr) -> Degrees to Radians2/1
  Rudder command  gradient1/1 -> Product3/1
  Product3/1 -> Sum3/2
  Lookup Table1/1 -> Product3/2
  [qbar_ps] -> Lookup Table1/1
  1.5/1 -> Switch/2
  Lookup Table2/1 -> Product4/1
  Product4/1 -> Sum5/1
  Abs/1 -> Lookup Table2/1
  Degrees to Radians2/1 -> dr (rad)/1
  Radians to Degrees/1 -> Transfer Fcn1/1, Abs/1
  Radians to Degrees1/1 -> Transfer Fcn4/1

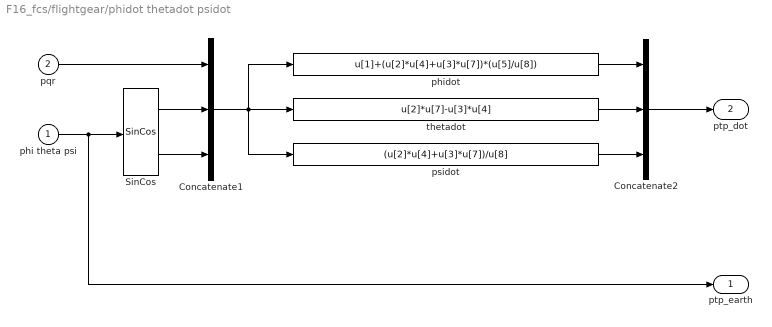
== system F16_fcs/flightgear/phidot thetadot psidot ==
  phi theta psi : Inport  OutDataType=sfix(16)  OutScaling=2^0
  pqr : Inport  Port=2  OutDataType=sfix(16)  OutScaling=2^0
  Concatenate1 : Concatenate  NumInputs=3  Mode=Vector
  Concatenate2 : Concatenate  NumInputs=3  Mode=Vector
  SinCos : aerolibutil/SinCos  SystemSampleTime=-1
  phidot : Fcn  Expr=u[1]+(u[2]*u[4]+u[3]*u[7])*(u[5]/u[8])
  psidot : Fcn  Expr=(u[2]*u[4]+u[3]*u[7])/u[8]
  thetadot : Fcn  Expr=u[2]*u[7]-u[3]*u[4]
  ptp_earth : Outport  OutDataType=sfix(16)  OutScaling=2^0
  ptp_dot : Outport  Port=2  OutDataType=sfix(16)  OutScaling=2^0
  wires:
  Concatenate1/1 -> psidot/1, phidot/1, thetadot/1
  pqr/1 -> Concatenate1/1
  phi theta psi/1 -> SinCos/1, ptp_earth/1
  psidot/1 -> Concatenate2/3
  thetadot/1 -> Concatenate2/2
  phidot/1 -> Concatenate2/1
  Concatenate2/1 -> ptp_dot/1
  SinCos/1 -> Concatenate1/2
  SinCos/2 -> Concatenate1/3

== system F16_fcs/flightgear/quaternions to Euler ==
  q : Inport
  Quaternions to Rotation Angles : aerolibtransform2/Quaternions to Rotation Angles  SystemSampleTime=-1  rotationOrder=ZYX
  Selector : Selector  InputPortWidth=3  IndexOptions=Index vector (dialog)  Indices=[3 2 1]  OutputSizes=1
  E : Outport
  wires:
  Quaternions to Rotation Angles/1 -> Selector/1
  q/1 -> Quaternions to Rotation Angles/1
  Selector/1 -> E/1

== system F16_fcs/sensors/quaternions to Euler ==
  q : Inport
  Quaternions to Rotation Angles : aerolibtransform2/Quaternions to Rotation Angles  SystemSampleTime=-1  rotationOrder=ZYX
  Selector : Selector  InputPortWidth=3  IndexOptions=Index vector (dialog)  Indices=[3 2 1]  OutputSizes=1
  E : Outport
  wires:
  Quaternions to Rotation Angles/1 -> Selector/1
  q/1 -> Quaternions to Rotation Angles/1
  Selector/1 -> E/1

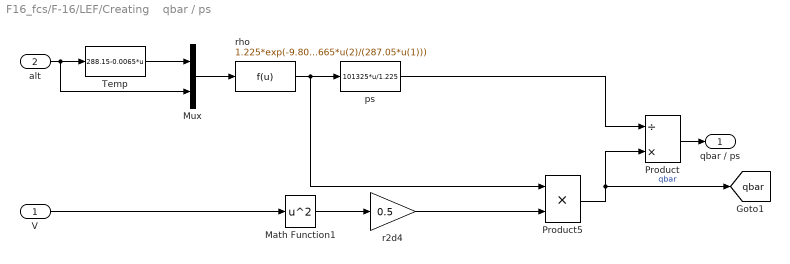
== system F16_fcs/F-16/LEF/Creating    qbar / ps ==
  V : Inport  OutDataType=sfix(16)  OutScaling=2^0
  alt : Inport  Port=2  OutDataType=sfix(16)  OutScaling=2^0
  Math Function1 : Math  Operator=square  OutDataType=sfix(16)  OutScaling=2^0  SaturateOnIntegerOverflow=on
  Mux : Mux  Inputs=2
  Product : Product  Inputs=/*  OutDataType=sfix(16)  OutScaling=2^0  SaturateOnIntegerOverflow=on  InputSameDT=on  OutDataTypeStr=Inherit: Same as first input
  Product5 : Product  Inputs=**  OutDataType=sfix(16)  OutScaling=2^0  SaturateOnIntegerOverflow=on  InputSameDT=on  OutDataTypeStr=Inherit: Same as first input
  Temp : Fcn  Expr=288.15-0.0065*u
  ps : Fcn  Expr=101325*u/1.225
  r2d4 : Gain  Gain=0.5  ParameterDataType=sfix(16)  ParameterScaling=2^0  OutDataType=sfix(16)  OutScaling=2^0  SaturateOnIntegerOverflow=on  OutDataTypeStr=Inherit: Same as input  ParamDataTypeStr=Inherit: Same as input
  rho : Fcn  Expr=1.225*exp(-9.80665*u(2)/(287.05*u(1)))
  qbar / ps : Outport  OutDataType=sfix(16)  OutScaling=2^0
  tag scope: qbar=global
  wires:
  ps/1 -> Product/1
  rho/1 -> Product5/1, ps/1
  Mux/1 -> rho/1
  Temp/1 -> Mux/1
  alt/1 -> Mux/2, Temp/1
  Math Function1/1 -> r2d4/1
  r2d4/1 -> Product5/2
  Product5/1 -> Product/2, [qbar]  "qbar"
  Product/1 -> qbar / ps/1
  V/1 -> Math Function1/1

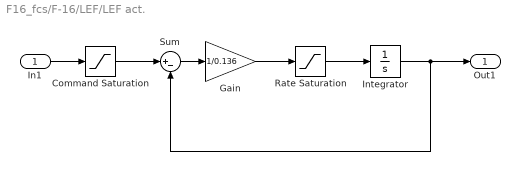
== system F16_fcs/F-16/LEF/LEF act. ==
  In1 : Inport  OutDataType=sfix(16)  OutScaling=2^0
  Command Saturation : Saturate  UpperLimit=25  LowerLimit=0
  Gain : Gain  Gain=1/0.136  ParameterDataType=sfix(16)  ParameterScaling=2^0  OutDataType=sfix(16)  OutScaling=2^0  SaturateOnIntegerOverflow=on  OutDataTypeStr=Inherit: Same as input  ParamDataTypeStr=Inherit: Same as input
  "Integrator " : Integrator  InitialCondition=dlef_trim*180/pi  UpperSaturationLimit=25  LowerSaturationLimit=-25
  Rate Saturation : Saturate  UpperLimit=25  LowerLimit=-25
  Sum : Sum  Inputs=|+-  OutDataType=sfix(16)  OutScaling=2^0  SaturateOnIntegerOverflow=on  InputSameDT=on  OutDataTypeStr=Inherit: Same as first input
  Out1 : Outport  OutDataType=sfix(16)  OutScaling=2^0
  wires:
  "Integrator "/1 -> Sum/2, Out1/1
  Rate Saturation/1 -> "Integrator "/1
  Gain/1 -> Rate Saturation/1
  Sum/1 -> Gain/1
  Command Saturation/1 -> Sum/1
  In1/1 -> Command Saturation/1

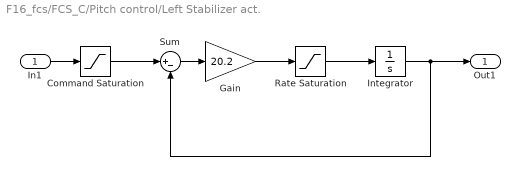
== system F16_fcs/FCS_C/Pitch control/Left Stabilizer act. ==
  In1 : Inport  OutDataType=sfix(16)  OutScaling=2^0
  Command Saturation : Saturate  UpperLimit=25  LowerLimit=-25
  Gain : Gain  Gain=20.2  ParameterDataType=sfix(16)  ParameterScaling=2^0  OutDataType=sfix(16)  OutScaling=2^0  SaturateOnIntegerOverflow=on  OutDataTypeStr=Inherit: Same as input  ParamDataTypeStr=Inherit: Same as input
  "Integrator " : Integrator  InitialCondition=der_trim  UpperSaturationLimit=25  LowerSaturationLimit=-25
  Rate Saturation : Saturate  UpperLimit=60  LowerLimit=-60
  Sum : Sum  Inputs=|+-  OutDataType=sfix(16)  OutScaling=2^0  SaturateOnIntegerOverflow=on  InputSameDT=on  OutDataTypeStr=Inherit: Same as first input
  Out1 : Outport  OutDataType=sfix(16)  OutScaling=2^0
  wires:
  In1/1 -> Command Saturation/1
  Command Saturation/1 -> Sum/1
  Sum/1 -> Gain/1
  Gain/1 -> Rate Saturation/1
  Rate Saturation/1 -> "Integrator "/1
  "Integrator "/1 -> Out1/1, Sum/2

== system F16_fcs/FCS_C/Pitch control/Right Stabilizer act. ==
  In1 : Inport  OutDataType=sfix(16)  OutScaling=2^0
  Command Saturation : Saturate  UpperLimit=25  LowerLimit=-25
  Gain : Gain  Gain=20.2  ParameterDataType=sfix(16)  ParameterScaling=2^0  OutDataType=sfix(16)  OutScaling=2^0  SaturateOnIntegerOverflow=on  OutDataTypeStr=Inherit: Same as input  ParamDataTypeStr=Inherit: Same as input
  "Integrator " : Integrator  InitialCondition=del_trim  UpperSaturationLimit=25  LowerSaturationLimit=-25
  Rate Saturation : Saturate  UpperLimit=60  LowerLimit=-60
  Sum : Sum  Inputs=|+-  OutDataType=sfix(16)  OutScaling=2^0  SaturateOnIntegerOverflow=on  InputSameDT=on  OutDataTypeStr=Inherit: Same as first input
  Out1 : Outport  OutDataType=sfix(16)  OutScaling=2^0
  wires:
  In1/1 -> Command Saturation/1
  Command Saturation/1 -> Sum/1
  Sum/1 -> Gain/1
  Gain/1 -> Rate Saturation/1
  Rate Saturation/1 -> "Integrator "/1
  "Integrator "/1 -> Out1/1, Sum/2

== system F16_fcs/FCS_C/Roll control/aileron actuator model ==
  da_c : Inport  OutDataType=sfix(16)  OutScaling=2^0
  Command Saturation : Saturate  UpperLimit=21.5  LowerLimit=-21.5
  Gain : Gain  Gain=20.2  ParameterDataType=sfix(16)  ParameterScaling=2^0  OutDataType=sfix(16)  OutScaling=2^0  SaturateOnIntegerOverflow=on  OutDataTypeStr=Inherit: Same as input  ParamDataTypeStr=Inherit: Same as input
  "Integrator " : Integrator  InitialCondition=da_trim  UpperSaturationLimit=25  LowerSaturationLimit=-25
  Rate Saturation : Saturate  UpperLimit=80  LowerLimit=-80
  Sum2 : Sum  Inputs=|+-  OutDataType=sfix(16)  OutScaling=2^0  SaturateOnIntegerOverflow=on  InputSameDT=on  OutDataTypeStr=Inherit: Same as first input
  da : Outport  OutDataType=sfix(16)  OutScaling=2^0
  wires:
  "Integrator "/1 -> Sum2/2, da/1
  Rate Saturation/1 -> "Integrator "/1
  Gain/1 -> Rate Saturation/1
  Sum2/1 -> Gain/1
  Command Saturation/1 -> Sum2/1
  da_c/1 -> Command Saturation/1

== system F16_fcs/FCS_C/Yaw control/rudder actuator model ==
  dr_c : Inport  OutDataType=sfix(16)  OutScaling=2^0
  Command Saturation : Saturate  UpperLimit=30  LowerLimit=-30
  Gain : Gain  Gain=20.2  ParameterDataType=sfix(16)  ParameterScaling=2^0  OutDataType=sfix(16)  OutScaling=2^0  SaturateOnIntegerOverflow=on  OutDataTypeStr=Inherit: Same as input  ParamDataTypeStr=Inherit: Same as input
  "Integrator " : Integrator  InitialCondition=dr_trim  UpperSaturationLimit=25  LowerSaturationLimit=-25
  Rate Saturation : Saturate  UpperLimit=120  LowerLimit=-120
  Sum2 : Sum  Inputs=|+-  OutDataType=sfix(16)  OutScaling=2^0  SaturateOnIntegerOverflow=on  InputSameDT=on  OutDataTypeStr=Inherit: Same as first input
  dr : Outport  OutDataType=sfix(16)  OutScaling=2^0
  wires:
  "Integrator "/1 -> Sum2/2, dr/1
  Rate Saturation/1 -> "Integrator "/1
  Gain/1 -> Rate Saturation/1
  Sum2/1 -> Gain/1
  Command Saturation/1 -> Sum2/1
  dr_c/1 -> Command Saturation/1
